simulink model "s3_21"  (Simulink 6.6)
settings: Solver=FixedStepDiscrete  StartTime=0.0  StopTime=t_d  FixedStep=Tc  MaxStep=Tc  RelTol=1e-6  AbsTol=1e-6
values from neighbouring files (symbols this model uses):
  a = [0.5; 0.3; 0.3]    [i3_21.m]
  Dq = 1e-6    (= 1e-06)    [i3_21.m]
  k_a = 35    [i3_21.m]
  K_p = diag([500,500])    [i3_21.m]
  q_i = inv_k3u(a,[p_i;phi_i])    [i3_21.m]
  Tc = 0.001    [i3_21.m]
  Ts = Tc    (= 0.001)    [i3_21.m]
undefined symbols (not defined in the file or in its folder): DiscIntNeverNeededParam
settings Model: Creator=luigivillani  LastModifiedBy=luigivillani  ExtModeAutoUpdateStatusClock=off
settings DataIOCC: LimitDataPoints=off  SaveOutput=off  SaveTime=off
settings OptimizationCC: BlockReduction=off  BooleanDataType=off
settings DebuggingCC: SignalResolutionControl=TryResolveAllWithWarning  SolverPrmCheckMsg=none  MultiTaskDSMMsg=warning  MultiTaskCondExecSysMsg=none  StrictBusMsg=None
settings HardwareCC: TargetUnknown=on
settings RTWCC: IncludeERTFirstTime=on

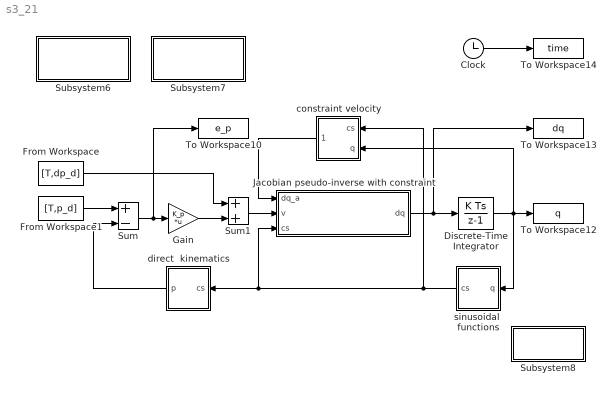
== system s3_21 ==
  Clock : Clock
  Discrete-Time Integrator : DiscreteIntegrator  InitialCondition=q_i  SampleTime=Tc  ICPrevOutput=DiscIntNeverNeededParam  ICPrevScaledInput=DiscIntNeverNeededParam
  From Workspace : FromWorkspace  VariableName=[T,dp_d]  SampleTime=Tc
  From Workspace1 : FromWorkspace  VariableName=[T,p_d]  SampleTime=Tc
  Gain : Gain  Gain=K_p  Multiplication=Matrix(K*u)  SampleTime=Tc
      mask Display: disp('K_p')
  Jacobian pseudo-inverse with constraint : Subsystem
      mask Display: disp('dag(J_p(q))dp + P(q)dq_a')
  Subsystem6 : Subsystem
      settings: OpenFcn=clear all;c = 0;i3_21;
      mask Display: disp('unconstrained\nsolution')
  Subsystem7 : Subsystem
      settings: OpenFcn=clear all;c=1;i3_21;
      mask Display: disp('constrained\nsolution')
  Subsystem8 : Subsystem  Orientation=left
      settings: OpenFcn=p3_21
      mask Display: disp('plot')
  Sum : Sum  Inputs=+-  SaturateOnIntegerOverflow=on  InputSameDT=on
  Sum1 : Sum  SaturateOnIntegerOverflow=on  InputSameDT=on
  To Workspace10 : ToWorkspace  VariableName=e_p  SampleTime=Ts  SaveFormat=Array
      settings: MaxDataPoints=2501
  To Workspace12 : ToWorkspace  VariableName=q  SampleTime=Ts  SaveFormat=Array
      settings: MaxDataPoints=2501
  To Workspace13 : ToWorkspace  VariableName=dq  SampleTime=Ts  SaveFormat=Array
      settings: MaxDataPoints=2501
  To Workspace14 : ToWorkspace  VariableName=time  SampleTime=Ts  SaveFormat=Array
      settings: MaxDataPoints=2501
  constraint velocity : Subsystem  Orientation=left
      mask Display: disp('dq_a')
  direct  kinematics : Subsystem  Orientation=left
      mask Display: disp('k_p(q)')
  sinusoidal  functions : Subsystem  Orientation=left
      mask Display: disp('cs(q)')
  wires:
  From Workspace1/1 -> Sum/1
  direct  kinematics/1(p) -> Sum/2
  Discrete-Time Integrator/1 -> To Workspace12/1, constraint velocity/2(q), sinusoidal  functions/1(q)
  sinusoidal  functions/1(cs) -> constraint velocity/1(cs), direct  kinematics/1(cs), Jacobian pseudo-inverse with constraint/3(cs)
  constraint velocity/1(dq_a) -> Jacobian pseudo-inverse with constraint/1(dq_a)
  Sum1/1 -> Jacobian pseudo-inverse with constraint/2(v)
  Clock/1 -> To Workspace14/1
  Jacobian pseudo-inverse with constraint/1(dq) -> To Workspace13/1, Discrete-Time Integrator/1
  From Workspace/1 -> Sum1/1
  Gain/1 -> Sum1/2
  Sum/1 -> To Workspace10/1, Gain/1

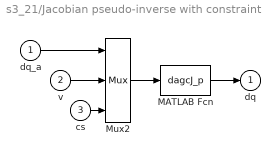
== system s3_21/Jacobian pseudo-inverse with constraint ==
  dq_a : Inport
  v : Inport  Port=2
  cs : Inport  Port=3
  MATLAB Fcn : MATLABFcn  MATLABFcn=dagcJ_p  OutputDimensions=3
      mask Display: disp('dagcJ_p')
  Mux2 : Mux  Inputs=[3,2,6]
  dq : Outport  InitialOutput=0
  wires:
  Mux2/1 -> MATLAB Fcn/1
  dq_a/1 -> Mux2/1
  MATLAB Fcn/1 -> dq/1
  v/1 -> Mux2/2
  cs/1 -> Mux2/3

== system s3_21/Subsystem6 ==
  note: start

== system s3_21/Subsystem7 ==
  note: start

== system s3_21/Subsystem8 ==
  note: start

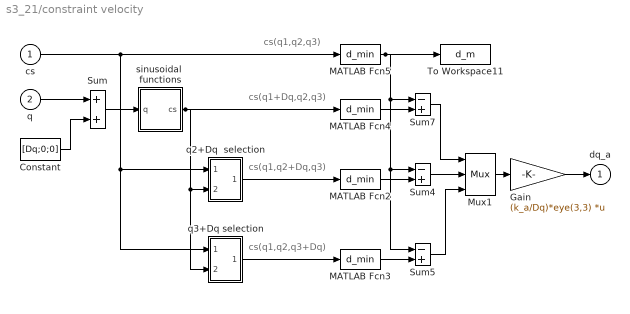
== system s3_21/constraint velocity ==
  note: cs(q1,q2,q3)
  note: cs(q1,q2,q3+Dq)
  note: cs(q1,q2+Dq,q3)
  note: cs(q1+Dq,q2,q3)
  cs : Inport
  q : Inport  Port=2
  Constant : Constant  Value=[Dq;0;0]
  Gain : Gain  Gain=(k_a/Dq)*eye(3,3)  Multiplication=Matrix(K*u)  SampleTime=Tc
      mask Display: disp('k_a/Dq')
  MATLAB Fcn{2..5} (4 alike) : MATLABFcn  MATLABFcn=d_min  OutputDimensions=1
      mask Display: disp('d_min')
  Mux1 : Mux  Inputs=3
  Sum : Sum  SaturateOnIntegerOverflow=on  InputSameDT=on
  Sum4 : Sum  Inputs=-+  SaturateOnIntegerOverflow=on  InputSameDT=on
  Sum5 : Sum  Inputs=-+  SaturateOnIntegerOverflow=on  InputSameDT=on
  Sum7 : Sum  Inputs=-+  SaturateOnIntegerOverflow=on  InputSameDT=on
  To Workspace11 : ToWorkspace  VariableName=d_m  SampleTime=Ts  SaveFormat=Array
      settings: MaxDataPoints=2501
  q2+Dq  selection : Subsystem
  q3+Dq selection : Subsystem
  sinusoidal  functions : Subsystem
      mask Display: disp('cs(q)')
  dq_a : Outport  InitialOutput=0
  wires:
  q2+Dq  selection/1(out_1) -> MATLAB Fcn2/1
  MATLAB Fcn2/1 -> Sum4/2
  MATLAB Fcn3/1 -> Sum5/2
  q/1 -> Sum/1
  Constant/1 -> Sum/2
  Sum/1 -> sinusoidal  functions/1(q)
  MATLAB Fcn4/1 -> Sum7/2
  q3+Dq selection/1(out_1) -> MATLAB Fcn3/1
  Sum4/1 -> Mux1/2
  Sum7/1 -> Mux1/1
  Sum5/1 -> Mux1/3
  Mux1/1 -> Gain/1
  Gain/1 -> dq_a/1
  MATLAB Fcn5/1 -> Sum5/1, Sum4/1, Sum7/1, To Workspace11/1
  sinusoidal  functions/1(cs) -> MATLAB Fcn4/1, q2+Dq  selection/2(cs_D), q3+Dq selection/2(cs_D)
  cs/1 -> MATLAB Fcn5/1, q2+Dq  selection/1(cs), q3+Dq selection/1(cs)

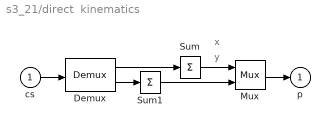
== system s3_21/direct  kinematics ==
  note: y
  note: x
  cs : Inport
  Demux : Demux  Outputs=[3,3]
  Mux : Mux  Inputs=2
  Sum : Sum  Inputs=+  SaturateOnIntegerOverflow=on  InputSameDT=on
  Sum1 : Sum  Inputs=+  SaturateOnIntegerOverflow=on  InputSameDT=on
  p : Outport  InitialOutput=0
  wires:
  Mux/1 -> p/1
  cs/1 -> Demux/1
  Demux/1 -> Sum/1
  Demux/2 -> Sum1/1
  Sum/1 -> Mux/1
  Sum1/1 -> Mux/2

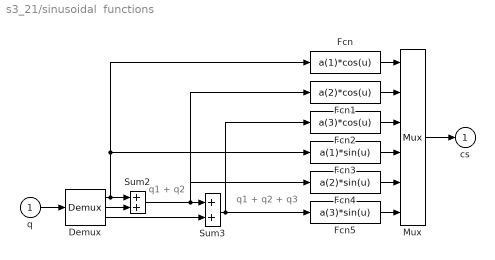
== system s3_21/sinusoidal  functions ==
  note: q1 + q2 + q3
  note: q1 + q2
  q : Inport
  Demux : Demux  Outputs=3
  Fcn : Fcn  Expr=a(1)*cos(u)
  Fcn1 : Fcn  Expr=a(2)*cos(u)
  Fcn2 : Fcn  Expr=a(3)*cos(u)
  Fcn3 : Fcn  Expr=a(1)*sin(u)
  Fcn4 : Fcn  Expr=a(2)*sin(u)
  Fcn5 : Fcn  Expr=a(3)*sin(u)
  Mux : Mux  Inputs=6
  Sum2 : Sum  SaturateOnIntegerOverflow=on  InputSameDT=on
  Sum3 : Sum  SaturateOnIntegerOverflow=on  InputSameDT=on
  cs : Outport  InitialOutput=0
  wires:
  Sum2/1 -> Sum3/1, Fcn1/1, Fcn4/1
  Sum3/1 -> Fcn2/1, Fcn5/1
  Demux/3 -> Sum3/2
  q/1 -> Demux/1
  Demux/2 -> Sum2/2
  Demux/1 -> Fcn/1, Fcn3/1, Sum2/1
  Mux/1 -> cs/1
  Fcn5/1 -> Mux/6
  Fcn4/1 -> Mux/5
  Fcn3/1 -> Mux/4
  Fcn2/1 -> Mux/3
  Fcn1/1 -> Mux/2
  Fcn/1 -> Mux/1

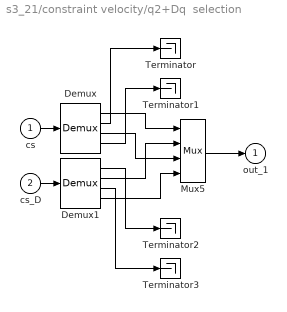
== system s3_21/constraint velocity/q2+Dq  selection ==
  cs : Inport
  cs_D : Inport  Port=2
  Demux : Demux  Outputs=[1,2,1,2]
  Demux1 : Demux  Outputs=[1,2,1,2]
  Mux5 : Mux  Inputs=[1,2,1,2]
  Terminator{,1..3} (4 alike) : Terminator
  out_1 : Outport  InitialOutput=0
  wires:
  cs/1 -> Demux/1
  Mux5/1 -> out_1/1
  cs_D/1 -> Demux1/1
  Demux1/2 -> Mux5/2
  Demux/1 -> Mux5/1
  Demux/3 -> Mux5/3
  Demux1/4 -> Mux5/4
  Demux/2 -> Terminator/1
  Demux/4 -> Terminator1/1
  Demux1/1 -> Terminator2/1
  Demux1/3 -> Terminator3/1

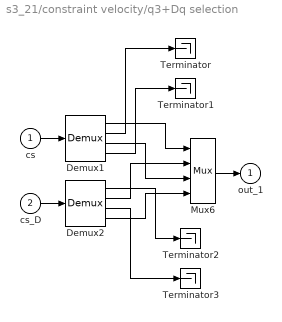
== system s3_21/constraint velocity/q3+Dq selection ==
  cs : Inport
  cs_D : Inport  Port=2
  Demux1 : Demux  Outputs=[2,1,2,1]
  Demux2 : Demux  Outputs=[2,1,2,1]
  Mux6 : Mux  Inputs=[2,1,2,1]
  Terminator{,1..3} (4 alike) : Terminator
  out_1 : Outport  InitialOutput=0
  wires:
  cs/1 -> Demux1/1
  Mux6/1 -> out_1/1
  cs_D/1 -> Demux2/1
  Demux1/1 -> Mux6/1
  Demux2/2 -> Mux6/2
  Demux1/3 -> Mux6/3
  Demux2/4 -> Mux6/4
  Demux1/2 -> Terminator/1
  Demux1/4 -> Terminator1/1
  Demux2/1 -> Terminator2/1
  Demux2/3 -> Terminator3/1

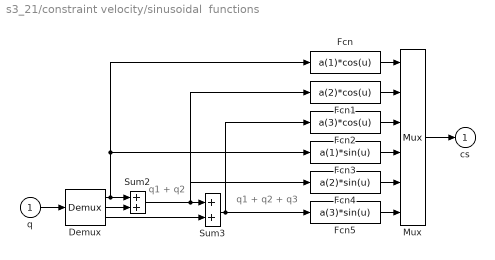
== system s3_21/constraint velocity/sinusoidal  functions ==
  note: q1 + q2
  note: q1 + q2 + q3
  q : Inport
  Demux : Demux  Outputs=3
  Fcn : Fcn  Expr=a(1)*cos(u)
  Fcn1 : Fcn  Expr=a(2)*cos(u)
  Fcn2 : Fcn  Expr=a(3)*cos(u)
  Fcn3 : Fcn  Expr=a(1)*sin(u)
  Fcn4 : Fcn  Expr=a(2)*sin(u)
  Fcn5 : Fcn  Expr=a(3)*sin(u)
  Mux : Mux  Inputs=6
  Sum2 : Sum  SaturateOnIntegerOverflow=on  InputSameDT=on
  Sum3 : Sum  SaturateOnIntegerOverflow=on  InputSameDT=on
  cs : Outport  InitialOutput=0
  wires:
  Fcn/1 -> Mux/1
  Fcn1/1 -> Mux/2
  Fcn2/1 -> Mux/3
  Fcn3/1 -> Mux/4
  Fcn4/1 -> Mux/5
  Fcn5/1 -> Mux/6
  Mux/1 -> cs/1
  Demux/2 -> Sum2/2
  q/1 -> Demux/1
  Demux/3 -> Sum3/2
  Sum2/1 -> Sum3/1, Fcn1/1, Fcn4/1
  Demux/1 -> Sum2/1, Fcn/1, Fcn3/1
  Sum3/1 -> Fcn5/1, Fcn2/1
